simulink model "svpwm_v1"  (R2017a)
settings: Solver=FixedStepAuto  StartTime=0.0  StopTime=50e-3  FixedStep=1/252000  MaxStep=1e-4  RelTol=1e-4
values from neighbouring files (symbols this model uses):
  Ts = (1/fs)    (= 0.00025)    [svpwm_param_v1.m]
libraries: powerlib x17, simulink x1, simulink_extras x1
settings Model: Creator=Shuvangkar  LastModifiedBy=Shuvangkar

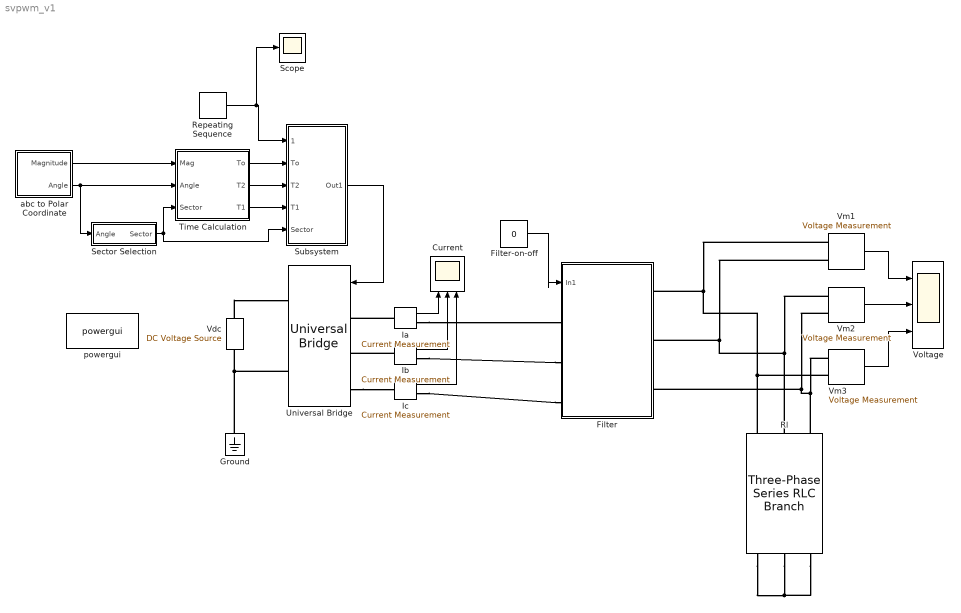
== system svpwm_v1 ==
  Current : Scope  NumInputPorts=3
  Filter : Subsystem
  Filter-on-off : Constant  Value=0
  Ground : powerlib/Elements/Ground  LConnTagsString=a
  Ia : powerlib/Measurements/Current Measurement  PhasorSimulation=off  OutputType=Complex  PSBequivalent=0
  Ib : powerlib/Measurements/Current Measurement  PhasorSimulation=off  OutputType=Complex  PSBequivalent=0
  Ic : powerlib/Measurements/Current Measurement  PhasorSimulation=off  OutputType=Complex  PSBequivalent=0
  Repeating Sequence : simulink/Sources/Repeating Sequence  rep_seq_t=[0 1/2 1]*(1/4000)  rep_seq_y=[0 1 0]
  Rl : powerlib/Elements/Three-Phase Series RLC Branch  LConnTagsString=A|B|C  RConnTagsString=A|B|C  BranchType=R  Resistance=10  Inductance=0  Capacitance=1e-6  Measurements=None
  Scope : Scope
  Sector Selection : Subsystem
  Subsystem : Subsystem
  Time Calculation : Subsystem
  Universal Bridge : powerlib/Power Electronics/Universal Bridge  Arms=3  SnubberResistance=1e5  SnubberCapacitance=inf  Device=IGBT / Diodes  Ron=1e-3  Lon=0  ForwardVoltages="[  0  0  ]"  ForwardVoltage=0  GTOparameters=[ 10e-6 , 20e-6 ]  IGBTparameters=[ 1e-6 , 2e-6 ]  Measurements=None  Measurements_2=None  converterType=Rectifier
  Vdc : powerlib/Electrical Sources/DC Voltage Source  Amplitude=600  Measurements=None
  Vm1 : powerlib/Measurements/Voltage Measurement  PhasorSimulation=off  OutputType=Complex  PSBequivalent=0
  Vm2 : powerlib/Measurements/Voltage Measurement  PhasorSimulation=off  OutputType=Complex  PSBequivalent=0
  Vm3 : powerlib/Measurements/Voltage Measurement  PhasorSimulation=off  OutputType=Complex  PSBequivalent=0
  Voltage : Scope  NumInputPorts=3
  abc to Polar Coordinate : Subsystem
  powergui : powerlib/powergui  Priority=1  SimulationMode=Discrete  SampleTime=1/252000  frequency=60  Iterations=50  frequencyindice=0  Pbase=100e6  ErrMax=1e-4  UnitsV=kV  UnitsW=MW  buscounter=0  FunctionMessages=off  echomessages=off  EnableUseOfTLC=off  CurrentSourceSwitches=off  DisableSnubberDevices=off  DisableRonSwitches=off  DisableVfSwitches=off  DisplayEquations=off  SolverType=Tustin/Backward Euler (TBE)  Interpol=off  ExternalGateDelay=off  methode=off  Ts=100  x0status=blocks  SPID=off  SwTol=0  HookPort=off  RestoreLinks=warning  ResistiveCurrentMeasurement=off  Frange=[0:2:500]  Ylog=off  Xlog=on  ShowGrid=off  save=off  variable=ZData  structure=0  ZoomFFT=off  StartTime=0.0  cycles=1  DisplayStyle=1  fundamental=60  FreqAxis=off  MaxFrequency=1000  frequencyindicesteady=1  RmsSteady=1  display=off
  wires:
  abc to Polar Coordinate/2(Angle) -> Time Calculation/2(Angle), Sector Selection/1(Angle)
  abc to Polar Coordinate/1(Magnitude) -> Time Calculation/1(Mag)
  Sector Selection/1(Sector) -> Time Calculation/3(Sector), Subsystem/5(Sector)
  Repeating Sequence/1 -> Scope/1, Subsystem/1(Repeatating Sequence)
  Time Calculation/1(To) -> Subsystem/2(To)
  Time Calculation/2(T2) -> Subsystem/3(T2)
  Time Calculation/3(T1) -> Subsystem/4(T1)
  Subsystem/1(Out1) -> Universal Bridge/1
  Ia/1 -> Current/1
  Ib/1 -> Current/2
  Ic/1 -> Current/3
  Vm2/1 -> Voltage/2
  Vm1/1 -> Voltage/1
  Vm3/1 -> Voltage/3
  Filter-on-off/1 -> Filter/1(In1)
  connections:
  Universal Bridge/RConn2 -- Vdc/LConn1 -- Ground/LConn1
  Vdc/RConn1 -- Universal Bridge/RConn1
  Ia/LConn1 -- Universal Bridge/LConn1
  Ib/LConn1 -- Universal Bridge/LConn2
  Universal Bridge/LConn3 -- Ic/LConn1
  Rl/LConn2 -- Vm1/LConn2 -- Filter/RConn2 -- Vm2/LConn1
  Rl/LConn3 -- Vm3/LConn1 -- Vm2/LConn2 -- Filter/RConn3
  Rl/RConn1 -- Rl/RConn3 -- Rl/RConn2
  Rl/LConn1 -- Vm3/LConn2 -- Vm1/LConn1 -- Filter/RConn1
  Ia/RConn1 -- Filter/LConn1
  Ib/RConn1 -- Filter/LConn2
  Ic/RConn1 -- Filter/LConn3

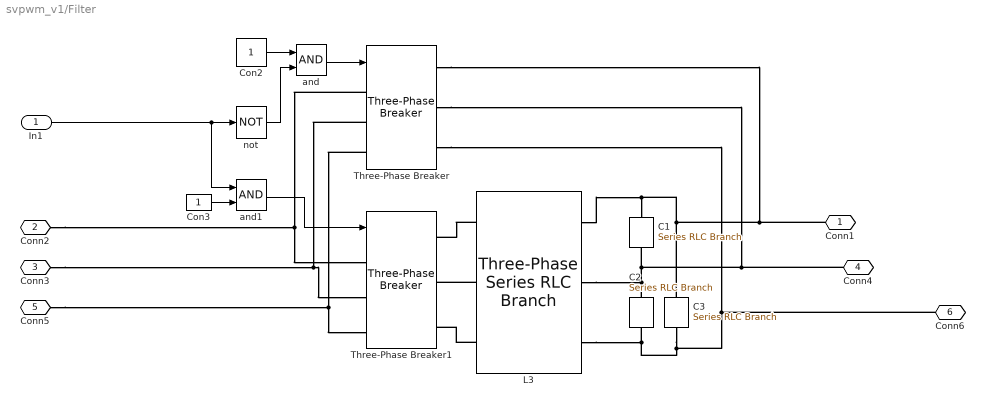
== system svpwm_v1/Filter ==
  In1 : Inport
  C1 : powerlib/Elements/Series RLC Branch  LConnTagsString=__new0  RConnTagsString=__new0  BranchType=C  Resistance=1  Inductance=1e-3  SetiL0=off  InitialCurrent=0  Capacitance=1e-6  Setx0=off  InitialVoltage=0  Measurements=None
  C2 : powerlib/Elements/Series RLC Branch  LConnTagsString=__new0  RConnTagsString=__new0  BranchType=C  Resistance=1  Inductance=1e-3  SetiL0=off  InitialCurrent=0  Capacitance=1e-6  Setx0=off  InitialVoltage=0  Measurements=None
  C3 : powerlib/Elements/Series RLC Branch  LConnTagsString=__new0  RConnTagsString=__new0  BranchType=C  Resistance=1  Inductance=1e-3  SetiL0=off  InitialCurrent=0  Capacitance=1e-6  Setx0=off  InitialVoltage=0  Measurements=None
  Con2 : Constant
  Con3 : Constant
  L3 : powerlib/Elements/Three-Phase Series RLC Branch  LConnTagsString=A|B|C  RConnTagsString=A|B|C  BranchType=L  Resistance=1  Inductance=1e-3  Capacitance=1e-6  Measurements=None
  Three-Phase Breaker : powerlib/Elements/Three-Phase Breaker  InitialState=open  SwitchA=on  SwitchB=on  SwitchC=on  SwitchTimes="[1/60  5/60]"  External=on  BreakerResistance=1e-6  SnubberResistance=1e6  SnubberCapacitance=inf  Measurements=None
  Three-Phase Breaker1 : powerlib/Elements/Three-Phase Breaker  InitialState=open  SwitchA=on  SwitchB=on  SwitchC=on  SwitchTimes="[1/60  5/60]"  External=on  BreakerResistance=0.01  SnubberResistance=1e6  SnubberCapacitance=inf  Measurements=None
  and : Logic  AllPortsSameDT=off  OutDataTypeStr=boolean
  and1 : Logic  AllPortsSameDT=off  OutDataTypeStr=boolean
  not : Logic  Operator=NOT  AllPortsSameDT=off  OutDataTypeStr=boolean
  Conn1 : PMIOPort  Port=1  Side=Right
  Conn2 : PMIOPort  Port=2  Side=Left
  Conn3 : PMIOPort  Port=3  Side=Left
  Conn4 : PMIOPort  Port=4  Side=Right
  Conn5 : PMIOPort  Port=5  Side=Left
  Conn6 : PMIOPort  Port=6  Side=Right
  wires:
  Con3/1 -> and1/2
  and/1 -> Three-Phase Breaker/1
  and1/1 -> Three-Phase Breaker1/1
  Con2/1 -> and/1
  In1/1 -> and1/1, not/1
  not/1 -> and/2
  connections:
  Three-Phase Breaker/LConn2 -- Conn3/RConn1 -- Three-Phase Breaker1/LConn2
  L3/LConn1 -- Three-Phase Breaker1/RConn1
  L3/LConn2 -- Three-Phase Breaker1/RConn2
  L3/LConn3 -- Three-Phase Breaker1/RConn3
  Three-Phase Breaker/LConn1 -- Conn2/RConn1 -- Three-Phase Breaker1/LConn1
  L3/RConn2 -- Conn4/RConn1 -- Three-Phase Breaker/RConn2 -- C1/RConn1 -- C2/LConn1
  L3/RConn3 -- Conn6/RConn1 -- Three-Phase Breaker/RConn3 -- C3/LConn1 -- C2/RConn1
  Three-Phase Breaker/LConn3 -- Conn5/RConn1 -- Three-Phase Breaker1/LConn3
  C3/RConn1 -- Conn1/RConn1 -- Three-Phase Breaker/RConn1 -- C1/LConn1 -- L3/RConn1

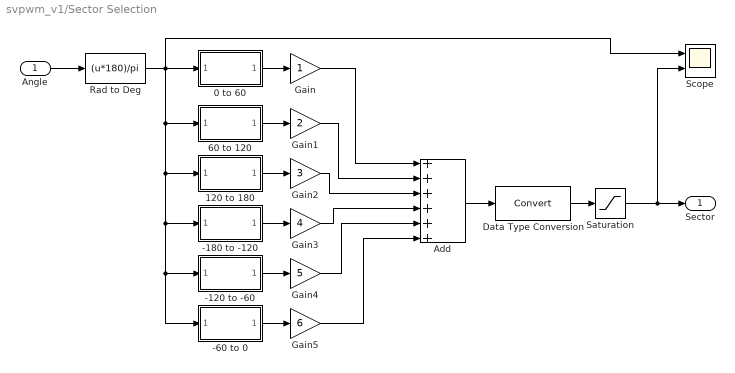
== system svpwm_v1/Sector Selection ==
  Angle : Inport
  -120 to -60 : Subsystem
  -180 to -120 : Subsystem
  -60 to 0 : Subsystem
  0 to 60 : Subsystem
  120 to 180 : Subsystem
  60 to 120 : Subsystem
  Add : Sum  Inputs=++++++
  Data Type Conversion : DataTypeConversion
  Gain : Gain
  Gain1 : Gain  Gain=2
  Gain2 : Gain  Gain=3
  Gain3 : Gain  Gain=4
  Gain4 : Gain  Gain=5
  Gain5 : Gain  Gain=6
  Rad to Deg : Fcn  Expr=(u*180)/pi
  Saturation : Saturate  UpperLimit=6  LowerLimit=1
  Scope : Scope  NumInputPorts=2
  Sector : Outport
  wires:
  Rad to Deg/1 -> Scope/1, -120 to -60/1(Angle), -60 to 0/1(Angle), -180 to -120/1(Angle), 120 to 180/1(Angle), 60 to 120/1(Angle), 0 to 60/1(Angle)
  Angle/1 -> Rad to Deg/1
  Gain4/1 -> Add/5
  0 to 60/1(sector) -> Gain/1
  60 to 120/1(sector) -> Gain1/1
  -120 to -60/1(sector) -> Gain4/1
  -180 to -120/1(sector) -> Gain3/1
  Gain5/1 -> Add/6
  -60 to 0/1(sector) -> Gain5/1
  Gain/1 -> Add/1
  120 to 180/1(sector) -> Gain2/1
  Gain1/1 -> Add/2
  Gain2/1 -> Add/3
  Gain3/1 -> Add/4
  Saturation/1 -> Scope/2, Sector/1
  Add/1 -> Data Type Conversion/1
  Data Type Conversion/1 -> Saturation/1

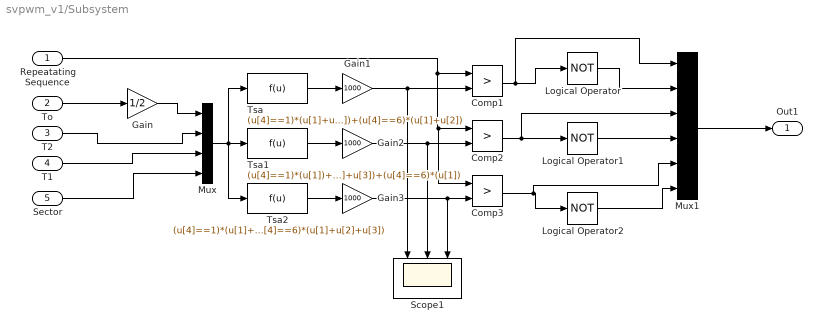
== system svpwm_v1/Subsystem ==
  Repeatating Sequence : Inport
  To : Inport  Port=2
  T2 : Inport  Port=3
  T1 : Inport  Port=4
  Sector : Inport  Port=5
  Comp1 : RelationalOperator  Operator=>  OutDataTypeStr=boolean  RndMeth=Simplest
  Comp2 : RelationalOperator  Operator=>  OutDataTypeStr=boolean  RndMeth=Simplest
  Comp3 : RelationalOperator  Operator=>  OutDataTypeStr=boolean  RndMeth=Simplest
  Gain : Gain  Gain=1/2
  Gain1 : Gain  Gain=1000
  Gain2 : Gain  Gain=1000
  Gain3 : Gain  Gain=1000
  Logical Operator : Logic  Operator=NOT  AllPortsSameDT=off  OutDataTypeStr=boolean
  Logical Operator1 : Logic  Operator=NOT  AllPortsSameDT=off  OutDataTypeStr=boolean
  Logical Operator2 : Logic  Operator=NOT  AllPortsSameDT=off  OutDataTypeStr=boolean
  Mux : Mux
  Mux1 : Mux  Inputs=6
  Scope1 : Scope  NumInputPorts=3
  Tsa : Fcn  Expr=(u[4]==1)*(u[1]+u[2]+u[3])+(u[4]==2)*(u[1]+u[2]+u[3])+(u[4]==3)*(u[1]+u[3])+(u[4]==4)*(u[1])+(u[4]==5)*(u[1])+(u[4]==6)*(u[1]+u[2])
  Tsa1 : Fcn  Expr=(u[4]==1)*(u[1])+(u[4]==2)*(u[1]+u[2])+(u[4]==3)*(u[1]+u[2]+u[3])+(u[4]==4)*(u[1]+u[2]+u[3])+(u[4]==5)*(u[1]+u[3])+(u[4]==6)*(u[1])
  Tsa2 : Fcn  Expr=(u[4]==1)*(u[1]+u[3])+(u[4]==2)*(u[1])+(u[4]==3)*(u[1])+(u[4]==4)*(u[1]+u[2])+(u[4]==5)*(u[1]+u[2]+u[3])+(u[4]==6)*(u[1]+u[2]+u[3])
  Out1 : Outport
  wires:
  Sector/1 -> Mux/4
  Mux/1 -> Tsa2/1, Tsa1/1, Tsa/1
  To/1 -> Gain/1
  Gain/1 -> Mux/1
  Tsa/1 -> Gain1/1
  T2/1 -> Mux/2
  T1/1 -> Mux/3
  Tsa1/1 -> Gain2/1
  Mux1/1 -> Out1/1
  Tsa2/1 -> Gain3/1
  Gain2/1 -> Scope1/2, Comp2/2
  Logical Operator2/1 -> Mux1/6
  Gain3/1 -> Scope1/3, Comp3/2
  Comp1/1 -> Mux1/1, Logical Operator/1
  Comp3/1 -> Mux1/5, Logical Operator2/1
  Repeatating Sequence/1 -> Comp3/1, Comp2/1, Comp1/1
  Comp2/1 -> Mux1/3, Logical Operator1/1
  Logical Operator/1 -> Mux1/2
  Logical Operator1/1 -> Mux1/4
  Gain1/1 -> Scope1/1, Comp1/2

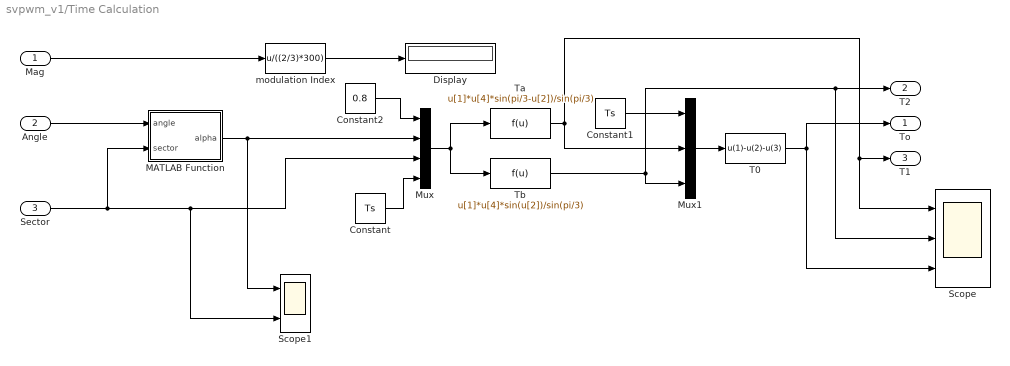
== system svpwm_v1/Time Calculation ==
  Mag : Inport
  Angle : Inport  Port=2
  Sector : Inport  Port=3
  Constant : Constant  Value=Ts
  Constant1 : Constant  Value=Ts
  Constant2 : Constant  Value=0.8
  Display : Display
  MATLAB Function : MATLAB Function  TreatAsAtomicUnit=on
  Mux : Mux
  Mux1 : Mux  Inputs=3
  Scope : Scope  NumInputPorts=3
  Scope1 : Scope  NumInputPorts=2
  T0 : Fcn  Expr=u(1)-u(2)-u(3)
  Ta : Fcn  Expr=u[1]*u[4]*sin(pi/3-u[2])/sin(pi/3)
  Tb : Fcn  Expr=u[1]*u[4]*sin(u[2])/sin(pi/3)
  modulation Index : Fcn  Expr=u/((2/3)*300)
  To : Outport
  T2 : Outport  Port=2
  T1 : Outport  Port=3
  wires:
  Mux1/1 -> T0/1
  modulation Index/1 -> Display/1
  Constant/1 -> Mux/4
  Ta/1 -> Scope/1, T1/1, Mux1/2
  T0/1 -> Scope/3, To/1
  Tb/1 -> Scope/2, T2/1, Mux1/3
  Mux/1 -> Tb/1, Ta/1
  Sector/1 -> MATLAB Function/2(sector), Scope1/2, Mux/3
  Constant1/1 -> Mux1/1
  Mag/1 -> modulation Index/1
  Constant2/1 -> Mux/1
  MATLAB Function/1(alpha) -> Scope1/1, Mux/2
  Angle/1 -> MATLAB Function/1(angle)

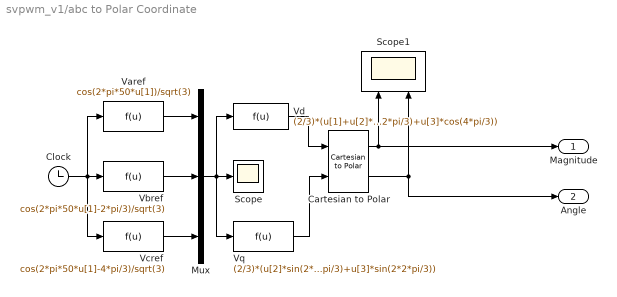
== system svpwm_v1/abc to Polar Coordinate ==
  Cartesian to Polar : simulink_extras/Transformations/Cartesian to Polar
      settings: SourceProductName=Simulink
  Clock : Clock
  Mux : Mux  Inputs=3
  Scope : Scope
  Scope1 : Scope  NumInputPorts=2
  Varef : Fcn  Expr=cos(2*pi*50*u[1])/sqrt(3)
  Vbref : Fcn  Expr=cos(2*pi*50*u[1]-2*pi/3)/sqrt(3)
  Vcref : Fcn  Expr=cos(2*pi*50*u[1]-4*pi/3)/sqrt(3)
  Vd : Fcn  Expr=(2/3)*(u[1]+u[2]*cos(2*pi/3)+u[3]*cos(4*pi/3))
  Vq : Fcn  Expr=(2/3)*(u[2]*sin(2*pi/3)+u[3]*sin(2*2*pi/3))
  Magnitude : Outport
  Angle : Outport  Port=2
  wires:
  Mux/1 -> Vq/1, Vd/1, Scope/1
  Cartesian to Polar/2 -> Angle/1, Scope1/2
  Cartesian to Polar/1 -> Magnitude/1, Scope1/1
  Vcref/1 -> Mux/3
  Vq/1 -> Cartesian to Polar/2
  Varef/1 -> Mux/1
  Vd/1 -> Cartesian to Polar/1
  Clock/1 -> Vcref/1, Vbref/1, Varef/1
  Vbref/1 -> Mux/2

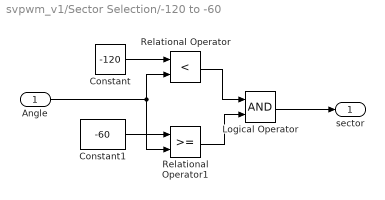
== system svpwm_v1/Sector Selection/-120 to -60 ==
  Angle : Inport
  Constant : Constant  Value=-120
  Constant1 : Constant  Value=-60
  Logical Operator : Logic  AllPortsSameDT=off  OutDataTypeStr=boolean
  Relational Operator : RelationalOperator  Operator=<  OutDataTypeStr=boolean  RndMeth=Simplest
  Relational Operator1 : RelationalOperator  OutDataTypeStr=boolean  RndMeth=Simplest
  sector : Outport
  wires:
  Relational Operator/1 -> Logical Operator/1
  Constant1/1 -> Relational Operator1/1
  Constant/1 -> Relational Operator/1
  Relational Operator1/1 -> Logical Operator/2
  Angle/1 -> Relational Operator/2, Relational Operator1/2
  Logical Operator/1 -> sector/1

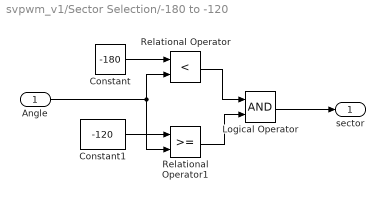
== system svpwm_v1/Sector Selection/-180 to -120 ==
  Angle : Inport
  Constant : Constant  Value=-180
  Constant1 : Constant  Value=-120
  Logical Operator : Logic  AllPortsSameDT=off  OutDataTypeStr=boolean
  Relational Operator : RelationalOperator  Operator=<  OutDataTypeStr=boolean  RndMeth=Simplest
  Relational Operator1 : RelationalOperator  OutDataTypeStr=boolean  RndMeth=Simplest
  sector : Outport
  wires:
  Relational Operator/1 -> Logical Operator/1
  Constant1/1 -> Relational Operator1/1
  Constant/1 -> Relational Operator/1
  Relational Operator1/1 -> Logical Operator/2
  Angle/1 -> Relational Operator/2, Relational Operator1/2
  Logical Operator/1 -> sector/1

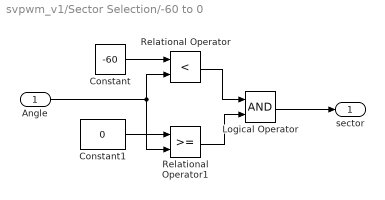
== system svpwm_v1/Sector Selection/-60 to 0 ==
  Angle : Inport
  Constant : Constant  Value=-60
  Constant1 : Constant  Value=0
  Logical Operator : Logic  AllPortsSameDT=off  OutDataTypeStr=boolean
  Relational Operator : RelationalOperator  Operator=<  OutDataTypeStr=boolean  RndMeth=Simplest
  Relational Operator1 : RelationalOperator  OutDataTypeStr=boolean  RndMeth=Simplest
  sector : Outport
  wires:
  Relational Operator/1 -> Logical Operator/1
  Constant1/1 -> Relational Operator1/1
  Constant/1 -> Relational Operator/1
  Relational Operator1/1 -> Logical Operator/2
  Angle/1 -> Relational Operator/2, Relational Operator1/2
  Logical Operator/1 -> sector/1

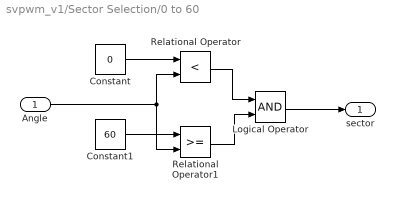
== system svpwm_v1/Sector Selection/0 to 60 ==
  Angle : Inport
  Constant : Constant  Value=0
  Constant1 : Constant  Value=60
  Logical Operator : Logic  AllPortsSameDT=off  OutDataTypeStr=boolean
  Relational Operator : RelationalOperator  Operator=<  OutDataTypeStr=boolean  RndMeth=Simplest
  Relational Operator1 : RelationalOperator  OutDataTypeStr=boolean  RndMeth=Simplest
  sector : Outport
  wires:
  Relational Operator/1 -> Logical Operator/1
  Constant1/1 -> Relational Operator1/1
  Constant/1 -> Relational Operator/1
  Relational Operator1/1 -> Logical Operator/2
  Angle/1 -> Relational Operator1/2, Relational Operator/2
  Logical Operator/1 -> sector/1

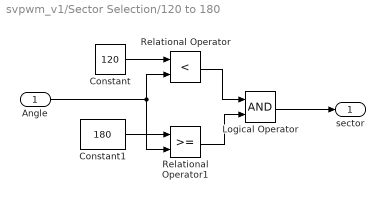
== system svpwm_v1/Sector Selection/120 to 180 ==
  Angle : Inport
  Constant : Constant  Value=120
  Constant1 : Constant  Value=180
  Logical Operator : Logic  AllPortsSameDT=off  OutDataTypeStr=boolean
  Relational Operator : RelationalOperator  Operator=<  OutDataTypeStr=boolean  RndMeth=Simplest
  Relational Operator1 : RelationalOperator  OutDataTypeStr=boolean  RndMeth=Simplest
  sector : Outport
  wires:
  Relational Operator/1 -> Logical Operator/1
  Constant1/1 -> Relational Operator1/1
  Constant/1 -> Relational Operator/1
  Relational Operator1/1 -> Logical Operator/2
  Angle/1 -> Relational Operator/2, Relational Operator1/2
  Logical Operator/1 -> sector/1

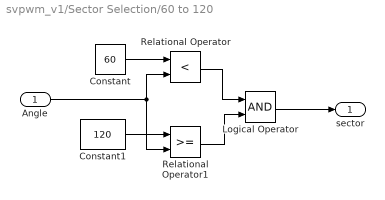
== system svpwm_v1/Sector Selection/60 to 120 ==
  Angle : Inport
  Constant : Constant  Value=60
  Constant1 : Constant  Value=120
  Logical Operator : Logic  AllPortsSameDT=off  OutDataTypeStr=boolean
  Relational Operator : RelationalOperator  Operator=<  OutDataTypeStr=boolean  RndMeth=Simplest
  Relational Operator1 : RelationalOperator  OutDataTypeStr=boolean  RndMeth=Simplest
  sector : Outport
  wires:
  Relational Operator/1 -> Logical Operator/1
  Constant1/1 -> Relational Operator1/1
  Constant/1 -> Relational Operator/1
  Relational Operator1/1 -> Logical Operator/2
  Angle/1 -> Relational Operator/2, Relational Operator1/2
  Logical Operator/1 -> sector/1

== matlab function svpwm_v1/Time Calculation/MATLAB Function ==
  data: angle input; alpha output; sector input
function alpha = fcn(angle,sector)
alpha = 0;
if (sector==1)
    alpha = angle;
elseif (sector==2)
    alpha = angle-pi/3;
elseif (sector == 3)
    alpha = angle- (2*pi/3);
elseif (sector==4)
    alpha = angle+pi;
elseif (sector==5)
    alpha = angle+(2*pi/3)
else 
    alpha = angle+pi/3;
end
